simulink model "Lab"  (R2023a)
settings: Solver=FixedStepAuto  StartTime=0.0  StopTime=10.0  FixedStep=0.001  RelTol=1e-3
settings Model: Creator=xiongj1  LastModifiedBy=xiongj1

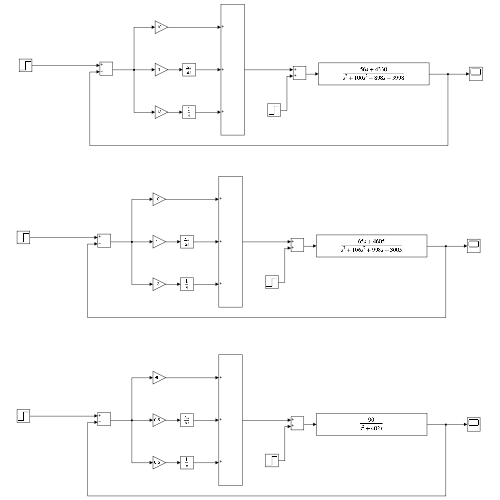
[thumbnail: Simulink's stored preview of the top-level diagram]
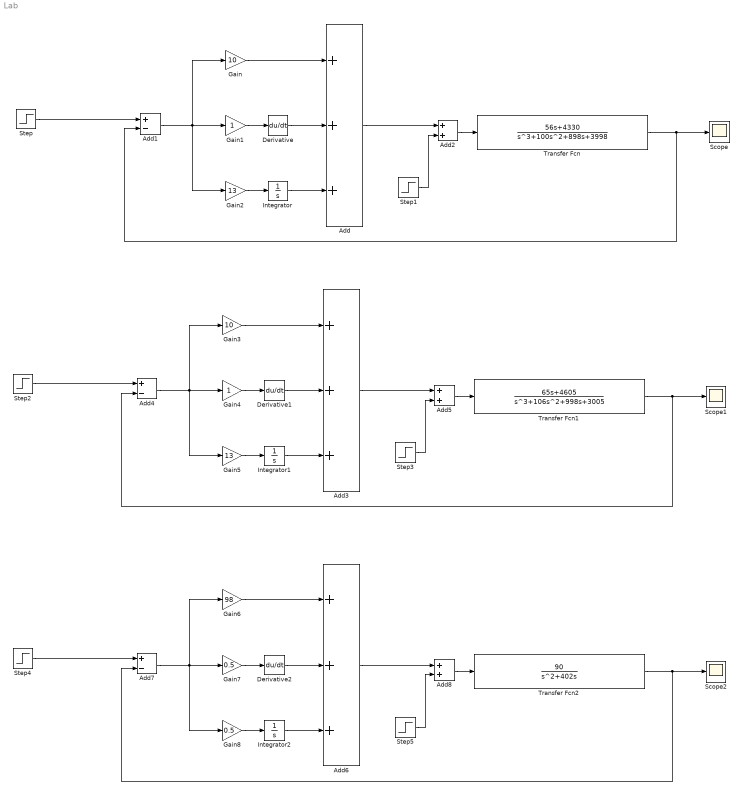
== system Lab ==
  Add : Sum  Inputs=+++
  Add1 : Sum  Inputs=+-
  Add2 : Sum
  Add3 : Sum  Inputs=+++
  Add4 : Sum  Inputs=+-
  Add5 : Sum
  Add6 : Sum  Inputs=+++
  Add7 : Sum  Inputs=+-
  Add8 : Sum
  Derivative : Derivative
  Derivative1 : Derivative
  Derivative2 : Derivative
  Gain : Gain  Gain=10
  Gain1 : Gain
  Gain2 : Gain  Gain=13
  Gain3 : Gain  Gain=10
  Gain4 : Gain
  Gain5 : Gain  Gain=13
  Gain6 : Gain  Gain=98
  Gain7 : Gain  Gain=0.5
  Gain8 : Gain  Gain=0.5
  Integrator : Integrator
  Integrator1 : Integrator
  Integrator2 : Integrator
  Scope : Scope
  Scope1 : Scope
  Scope2 : Scope
  Step : Step  Time=0  SampleTime=0
  Step1 : Step  Time=5  SampleTime=0
  Step2 : Step  Time=0  SampleTime=0
  Step3 : Step  Time=5  SampleTime=0
  Step4 : Step  Time=0  SampleTime=0
  Step5 : Step  Time=5  SampleTime=0
  Transfer Fcn : TransferFcn  Numerator=[56 4330]  Denominator=[1 100 898 3998]
  Transfer Fcn1 : TransferFcn  Numerator=[65 4605]  Denominator=[1 106 998 3005]
  Transfer Fcn2 : TransferFcn  Numerator=[90]  Denominator=[1 402 0]
  wires:
  Gain/1 -> Add/1
  Gain1/1 -> Derivative/1
  Gain2/1 -> Integrator/1
  Add1/1 -> Gain2/1, Gain1/1, Gain/1
  Step/1 -> Add1/1
  Transfer Fcn/1 -> Add1/2, Scope/1
  Add2/1 -> Transfer Fcn/1
  Add/1 -> Add2/1
  Derivative/1 -> Add/2
  Integrator/1 -> Add/3
  Step1/1 -> Add2/2
  Step3/1 -> Add5/2
  Integrator1/1 -> Add3/3
  Derivative1/1 -> Add3/2
  Add3/1 -> Add5/1
  Add5/1 -> Transfer Fcn1/1
  Transfer Fcn1/1 -> Scope1/1, Add4/2
  Step2/1 -> Add4/1
  Add4/1 -> Gain3/1, Gain4/1, Gain5/1
  Gain5/1 -> Integrator1/1
  Gain4/1 -> Derivative1/1
  Gain3/1 -> Add3/1
  Gain6/1 -> Add6/1
  Gain7/1 -> Derivative2/1
  Gain8/1 -> Integrator2/1
  Add7/1 -> Gain8/1, Gain7/1, Gain6/1
  Step4/1 -> Add7/1
  Transfer Fcn2/1 -> Add7/2, Scope2/1
  Add8/1 -> Transfer Fcn2/1
  Add6/1 -> Add8/1
  Derivative2/1 -> Add6/2
  Integrator2/1 -> Add6/3
  Step5/1 -> Add8/2
